simulink model "DESC_Model_2_RC"  (R2020b)
settings: Solver=VariableStepAuto  StartTime=0.0  StopTime=66747  RelTol=1e-3
undefined symbols (not defined in the file): g, M, OCV0, OCVRel, Q, R0cha, R0dch, R1, R2, RC1, RC2, T
settings Model: OrderedModelArguments=off  Creator=erhan  LastModifiedBy=erhan
settings DataIOCC: ReturnWorkspaceOutputs=off
settings DebuggingCC: ArithmeticOperatorsInVariantConditions=warning
settings SFSimCC: SimUseLocalCustomCode=off  CustomCodeUndefinedFunction=UseInterfaceOnly
settings RTWCC: RTWUseLocalCustomCode=off

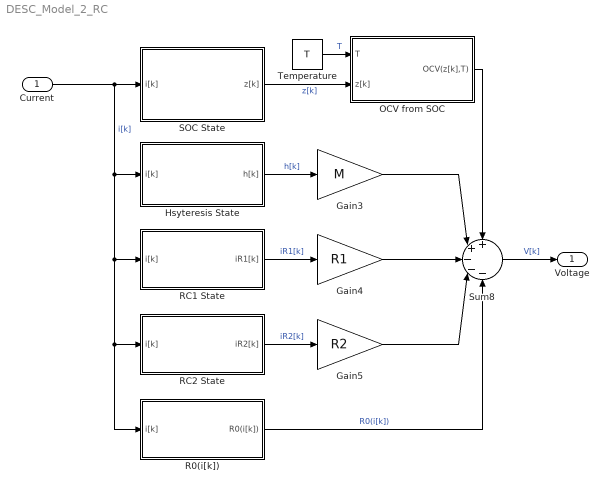
== system DESC_Model_2_RC ==
  Current : Inport
  Gain3 : Gain  Gain=M
  Gain4 : Gain  Gain=R1
  Gain5 : Gain  Gain=R2
  Hsyteresis State : Subsystem
  OCV from SOC : Subsystem
  R0(i[k]) : Subsystem
  RC1 State : Subsystem
  RC2 State : Subsystem
  SOC State : Subsystem
  Sum8 : Sum  Inputs=++---
  Temperature : Constant  Value=T
  Voltage : Outport  VectorParamsAs1DForOutWhenUnconnected=off
  wires:
  Gain4/1 -> Sum8/3
  Gain3/1 -> Sum8/2
  Gain5/1 -> Sum8/4
  SOC State/1(z[k]) -> OCV from SOC/2(z[k])  "z[k]"
  OCV from SOC/1(OCV(z[k],T)) -> Sum8/1
  Temperature/1 -> OCV from SOC/1(T)  "T"
  Hsyteresis State/1(h[k]) -> Gain3/1  "h[k]"
  RC1 State/1(iR1[k]) -> Gain4/1  "iR1[k]"
  RC2 State/1(iR2[k]) -> Gain5/1  "iR2[k]"
  R0(i[k])/1(R0(i[k])) -> Sum8/5  "R0(i[k])"
  Sum8/1 -> Voltage/1  "V[k]"
  Current/1 -> R0(i[k])/1(i[k]), RC2 State/1(i[k]), RC1 State/1(i[k]), Hsyteresis State/1(i[k]), SOC State/1(i[k])  "i[k]"

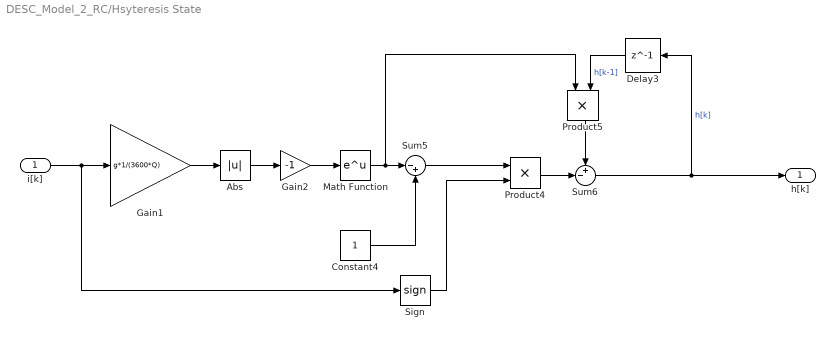
== system DESC_Model_2_RC/Hsyteresis State ==
  i[k] : Inport
  Abs : Abs
  Constant4 : Constant
  Delay3 : Delay  DelayLength=1  InitialCondition=-1  SampleTime=1
  Gain1 : Gain  Gain=g*1/(3600*Q)
  Gain2 : Gain  Gain=-1
  Math Function : Math  SignedPower=on  SaturateOnIntegerOverflow=on
  Product4 : Product
  Product5 : Product
  Sign : Signum
  Sum5 : Sum  Inputs=|-+
  Sum6 : Sum  Inputs=+-|
  h[k] : Outport
  wires:
  Delay3/1 -> Product5/2  "h[k-1]"
  Sum6/1 -> h[k]/1, Delay3/1  "h[k]"
  i[k]/1 -> Sign/1, Gain1/1
  Product5/1 -> Sum6/1
  Gain2/1 -> Math Function/1
  Math Function/1 -> Product5/1, Sum5/1
  Abs/1 -> Gain2/1
  Gain1/1 -> Abs/1
  Product4/1 -> Sum6/2
  Constant4/1 -> Sum5/2
  Sign/1 -> Product4/2
  Sum5/1 -> Product4/1

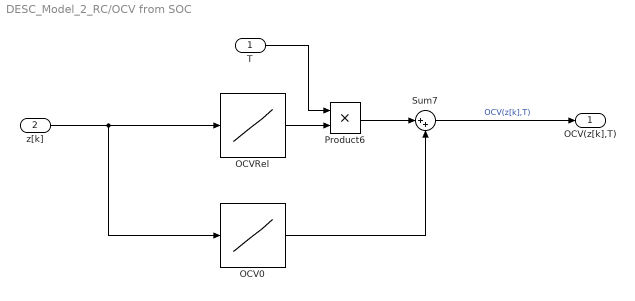
== system DESC_Model_2_RC/OCV from SOC ==
  T : Inport
  z[k] : Inport  Port=2
  OCV0 : Lookup_n-D  NumberOfTableDimensions=1  BreakpointsForDimension1=[0:0.005:1]  Table=OCV0  InternalRulePriority=Speed  RndMeth=Simplest  InputSameDT=on
  OCVRel : Lookup_n-D  NumberOfTableDimensions=1  BreakpointsForDimension1=[0:0.005:1]  Table=OCVRel  InternalRulePriority=Speed  RndMeth=Simplest  InputSameDT=on
  Product6 : Product
  Sum7 : Sum  Inputs=|++
  OCV(z[k],T) : Outport
  wires:
  OCVRel/1 -> Product6/2
  T/1 -> Product6/1
  Product6/1 -> Sum7/1
  Sum7/1 -> OCV(z[k],T)/1  "OCV(z[k],T)"
  z[k]/1 -> OCV0/1, OCVRel/1
  OCV0/1 -> Sum7/2

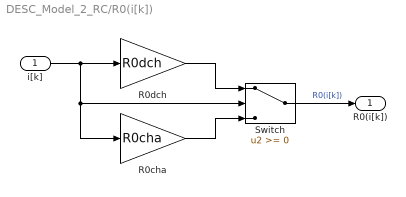
== system DESC_Model_2_RC/R0(i[k]) ==
  i[k] : Inport
  R0cha : Gain  Gain=R0cha
  R0dch : Gain  Gain=R0dch
  Switch : Switch
  R0(i[k]) : Outport
  wires:
  i[k]/1 -> R0cha/1, Switch/2, R0dch/1
  R0cha/1 -> Switch/3
  R0dch/1 -> Switch/1
  Switch/1 -> R0(i[k])/1  "R0(i[k])"

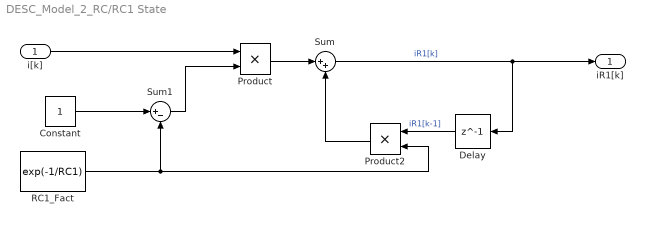
== system DESC_Model_2_RC/RC1 State ==
  i[k] : Inport
  Constant : Constant
  Delay : Delay  DelayLength=1  InitialCondition=0  SampleTime=1
  Product : Product
  Product2 : Product
  RC1_Fact : Constant  Value=exp(-1/RC1)
  Sum : Sum  Inputs=|++
  Sum1 : Sum  Inputs=|+-
  iR1[k] : Outport
  wires:
  Product/1 -> Sum/1
  i[k]/1 -> Product/1
  Constant/1 -> Sum1/1
  Sum/1 -> iR1[k]/1, Delay/1  "iR1[k]"
  RC1_Fact/1 -> Sum1/2, Product2/2
  Delay/1 -> Product2/1  "iR1[k-1]"
  Product2/1 -> Sum/2
  Sum1/1 -> Product/2

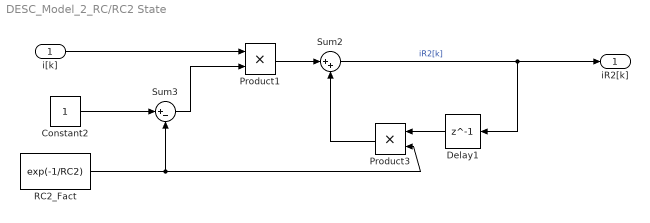
== system DESC_Model_2_RC/RC2 State ==
  i[k] : Inport
  Constant2 : Constant
  Delay1 : Delay  DelayLength=1  InitialCondition=0  SampleTime=1
  Product1 : Product
  Product3 : Product
  RC2_Fact : Constant  Value=exp(-1/RC2)
  Sum2 : Sum  Inputs=|++
  Sum3 : Sum  Inputs=|+-
  iR2[k] : Outport
  wires:
  i[k]/1 -> Product1/1
  Sum2/1 -> iR2[k]/1, Delay1/1  "iR2[k]"
  Delay1/1 -> Product3/1
  Sum3/1 -> Product1/2
  Product1/1 -> Sum2/1
  RC2_Fact/1 -> Product3/2, Sum3/2
  Constant2/1 -> Sum3/1
  Product3/1 -> Sum2/2

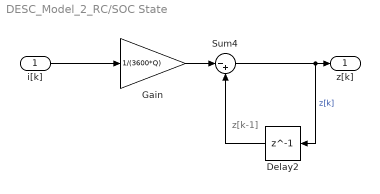
== system DESC_Model_2_RC/SOC State ==
  note: z[k-1]
  i[k] : Inport
  Delay2 : Delay  DelayLength=1  InitialCondition=1  SampleTime=1
  Gain : Gain  Gain=1/(3600*Q)
  Sum4 : Sum  Inputs=|-+
  z[k] : Outport
  wires:
  Gain/1 -> Sum4/1
  Sum4/1 -> Delay2/1, z[k]/1  "z[k]"
  Delay2/1 -> Sum4/2
  i[k]/1 -> Gain/1
